simulink model "ball"  (Simulink 4.00)
settings: Solver=ode45  StartTime=0.0  StopTime=10.0  RelTol=1e-2
settings Model: LastModifiedBy=hespanha  LimitDataPoints=off  ZeroCross=off  ExtModeTrigMode=oneshot  ExtModeArmWhenConnect=off  BlockReductionOpt=off

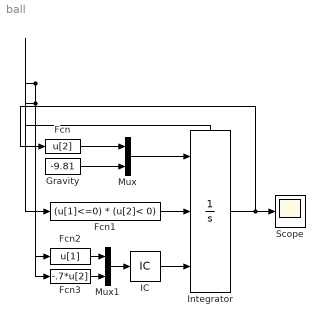
== system ball ==
  Fcn : Fcn  Expr=u[2]
  Fcn1 : Fcn  Expr=(u[1]<=0) * (u[2]< 0)
  Fcn2 : Fcn  Expr=u[1]
  Fcn3 : Fcn  Expr=-.7*u[2]
  Gravity : Constant  Value=-9.81
  IC : InitialCondition  Value=[10;5]
  Integrator : Integrator  ExternalReset=rising  InitialConditionSource=external  InitialCondition=0  LimitOutput=on  UpperSaturationLimit=inf  LowerSaturationLimit=[0;-inf]  ShowSaturationPort=off  ShowStatePort=on  AbsoluteTolerance=auto
  Mux : Mux  Inputs=2
  Mux1 : Mux  Inputs=2
  Scope : Scope
      settings: TimeRange=10  YMin=-15  YMax=15  SaveToWorkspace=off  SaveName=ScopeData  LimitDataPoints=on  MaxDataPoints=5000
  wires:
  Fcn1/1 -> Integrator/2
  Mux/1 -> Integrator/1
  Gravity/1 -> Mux/2
  Fcn/1 -> Mux/1
  Fcn3/1 -> Mux1/2
  Fcn2/1 -> Mux1/1
  Integrator/State -> Fcn1/1, Fcn2/1, Fcn3/1
  Mux1/1 -> IC/1
  IC/1 -> Integrator/3
  Integrator/1 -> Scope/1, Fcn/1
